simulink library "lib_IronAir"  (R2025b)
settings: Solver=VariableStepAuto  StartTime=0.0  StopTime=10.0  RelTol=1e-3
values from neighbouring files (symbols this model uses):
  IronAir = lib_IronAir_init_params_only()    [generate_mock_cell_curves.m]    (also in lib_IronAir.sldd = 0.01
                        5.0
                    
      ; lib_IronAir_init.m = struct())
undefined symbols (not defined in the file or in its folder): ironair_aggregate_vector, ironair_der_ride_through_vector, ironair_plant_schedule_vector, ironair_sl_cell_dydt, ironair_sl_cell_out, ironair_sl_cell_y0, ironair_sl_electrolyte_dydt, ironair_sl_h2_dydt, ironair_sl_h2_out, ironair_sl_metal_dydt, ironair_sl_metal_out, ironair_sl_oer_out, ironair_sl_orr_dydt, ironair_sl_orr_eta, ironair_sl_thermal_dydt, ironair_standards_assert_vector
settings Model: Creator=admin  LastModifiedBy=admin

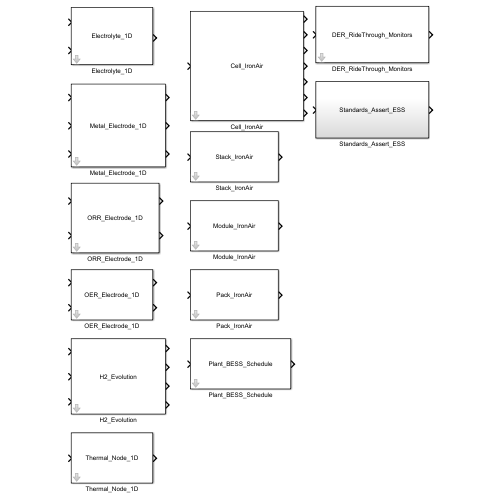
[thumbnail: Simulink's stored preview of the top-level diagram]
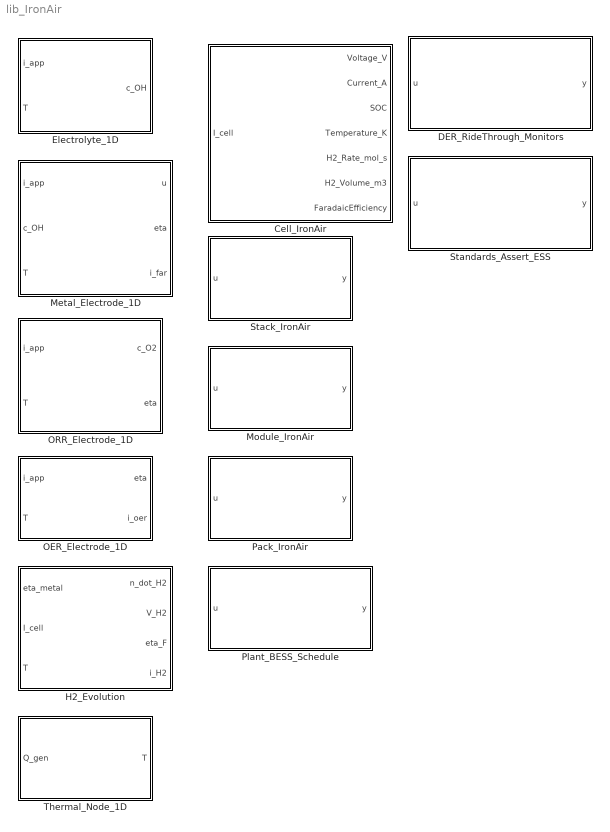
== system lib_IronAir ==
  Cell_IronAir : Subsystem  mask(IronAir){}
      mask help: Iron-Air first-order ODE block Cell_IronAir (Integrator + dy/dt). No S-Functions. Requirements: SSS009 IRS001 SRS017
      mask Help:
      | Continuous first-order ODE realization using Simulink Integrator.
      | Requirements: SSS009 IRS001 SRS017
      mask Display: fprintf('Cell_IronAir')
  DER_RideThrough_Monitors : Subsystem  mask(IronAir){}
      mask help: Iron-Air first-order ODE block DER_RideThrough_Monitors (Integrator + dy/dt). No S-Functions. Requirements: SSS012 SRS011 SRS013
      mask Help:
      | Continuous first-order ODE realization using Simulink Integrator.
      | Requirements: SSS012 SRS011 SRS013
      mask Display: fprintf('DER_RideThrough_Monitors')
  Electrolyte_1D : Subsystem  mask(IronAir){}
      mask help: Iron-Air first-order ODE block Electrolyte_1D (Integrator + dy/dt). No S-Functions. Requirements: SSS003 SRS003 SRS017
      mask Help:
      | Continuous first-order ODE realization using Simulink Integrator.
      | Requirements: SSS003 SRS003 SRS017
      mask Display: fprintf('Electrolyte_1D')
  H2_Evolution : Subsystem  mask(IronAir){}
      mask help: Iron-Air first-order ODE block H2_Evolution (Integrator + dy/dt). No S-Functions. Requirements: SSS007 SRS004 SRS017
      mask Help:
      | Continuous first-order ODE realization using Simulink Integrator.
      | Requirements: SSS007 SRS004 SRS017
      mask Display: fprintf('H2_Evolution')
  Metal_Electrode_1D : Subsystem  mask(IronAir){}
      mask help: Iron-Air first-order ODE block Metal_Electrode_1D (Integrator + dy/dt). No S-Functions. Requirements: SSS004 SRS002 SRS017
      mask Help:
      | Continuous first-order ODE realization using Simulink Integrator.
      | Requirements: SSS004 SRS002 SRS017
      mask Display: fprintf('Metal_Electrode_1D')
  Module_IronAir : Subsystem  mask(IronAir){}
      mask help: Iron-Air first-order ODE block Module_IronAir (Integrator + dy/dt). No S-Functions. Requirements: SSS010
      mask Help:
      | Continuous first-order ODE realization using Simulink Integrator.
      | Requirements: SSS010
      mask Display: fprintf('Module_IronAir')
  OER_Electrode_1D : Subsystem  mask(IronAir){}
      mask help: Iron-Air first-order ODE block OER_Electrode_1D (Integrator + dy/dt). No S-Functions. Requirements: SSS006 SRS002
      mask Help:
      | Continuous first-order ODE realization using Simulink Integrator.
      | Requirements: SSS006 SRS002
      mask Display: fprintf('OER_Electrode_1D')
  ORR_Electrode_1D : Subsystem  mask(IronAir){}
      mask help: Iron-Air first-order ODE block ORR_Electrode_1D (Integrator + dy/dt). No S-Functions. Requirements: SSS005 SRS002 SRS017
      mask Help:
      | Continuous first-order ODE realization using Simulink Integrator.
      | Requirements: SSS005 SRS002 SRS017
      mask Display: fprintf('ORR_Electrode_1D')
  Pack_IronAir : Subsystem  mask(IronAir){}
      mask help: Iron-Air first-order ODE block Pack_IronAir (Integrator + dy/dt). No S-Functions. Requirements: SSS010 IRS002
      mask Help:
      | Continuous first-order ODE realization using Simulink Integrator.
      | Requirements: SSS010 IRS002
      mask Display: fprintf('Pack_IronAir')
  Plant_BESS_Schedule : Subsystem  mask(IronAir){}
      mask help: Iron-Air first-order ODE block Plant_BESS_Schedule (Integrator + dy/dt). No S-Functions. Requirements: SSS011 SRS006
      mask Help:
      | Continuous first-order ODE realization using Simulink Integrator.
      | Requirements: SSS011 SRS006
      mask Display: fprintf('Plant_BESS_Schedule')
  Stack_IronAir : Subsystem  mask(IronAir){}
      mask help: Iron-Air first-order ODE block Stack_IronAir (Integrator + dy/dt). No S-Functions. Requirements: SSS010
      mask Help:
      | Continuous first-order ODE realization using Simulink Integrator.
      | Requirements: SSS010
      mask Display: fprintf('Stack_IronAir')
  Standards_Assert_ESS : Subsystem  mask(IronAir){}
      mask help: Iron-Air first-order ODE block Standards_Assert_ESS (Integrator + dy/dt). No S-Functions. Requirements: SSS013 SRS012 SRS014 SRS015
      mask Help:
      | Continuous first-order ODE realization using Simulink Integrator.
      | Requirements: SSS013 SRS012 SRS014 SRS015
      mask Display: fprintf('Standards_Assert_ESS')
  Thermal_Node_1D : Subsystem  mask(IronAir){}
      mask help: Iron-Air first-order ODE block Thermal_Node_1D (Integrator + dy/dt). No S-Functions. Requirements: SSS008 SRS007 SRS017
      mask Help:
      | Continuous first-order ODE realization using Simulink Integrator.
      | Requirements: SSS008 SRS007 SRS017
      mask Display: fprintf('Thermal_Node_1D')

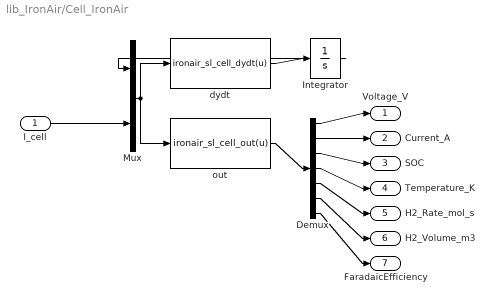
== system lib_IronAir/Cell_IronAir ==
  I_cell : Inport
  Demux : Demux  Outputs=7
  Integrator : Integrator  InitialCondition=ironair_sl_cell_y0()
  Mux : Mux  Inputs=2
  dydt : MATLABFcn  MATLABFcn=ironair_sl_cell_dydt(u)  OutputDimensions=13
  out : MATLABFcn  MATLABFcn=ironair_sl_cell_out(u)  OutputDimensions=7
  Voltage_V : Outport
  Current_A : Outport  Port=2
  SOC : Outport  Port=3
  Temperature_K : Outport  Port=4
  H2_Rate_mol_s : Outport  Port=5
  H2_Volume_m3 : Outport  Port=6
  FaradaicEfficiency : Outport  Port=7
  wires:
  Integrator/1 -> Mux/1
  I_cell/1 -> Mux/2
  Mux/1 -> dydt/1, out/1
  dydt/1 -> Integrator/1
  out/1 -> Demux/1
  Demux/1 -> Voltage_V/1
  Demux/2 -> Current_A/1
  Demux/3 -> SOC/1
  Demux/4 -> Temperature_K/1
  Demux/5 -> H2_Rate_mol_s/1
  Demux/6 -> H2_Volume_m3/1
  Demux/7 -> FaradaicEfficiency/1

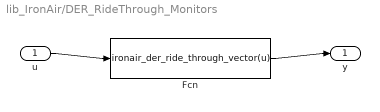
== system lib_IronAir/DER_RideThrough_Monitors ==
  u : Inport
  Fcn : MATLABFcn  MATLABFcn=ironair_der_ride_through_vector(u)  OutputDimensions=3
  y : Outport
  wires:
  u/1 -> Fcn/1
  Fcn/1 -> y/1

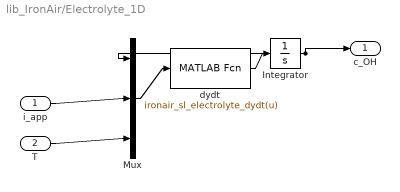
== system lib_IronAir/Electrolyte_1D ==
  i_app : Inport
  T : Inport  Port=2
  Integrator : Integrator  InitialCondition=IronAir.Electrolyte.c_init
  Mux : Mux  Inputs=3
  dydt : MATLABFcn  MATLABFcn=ironair_sl_electrolyte_dydt(u)  OutputDimensions=5
  c_OH : Outport
  wires:
  Integrator/1 -> Mux/1, c_OH/1
  i_app/1 -> Mux/2
  T/1 -> Mux/3
  Mux/1 -> dydt/1
  dydt/1 -> Integrator/1

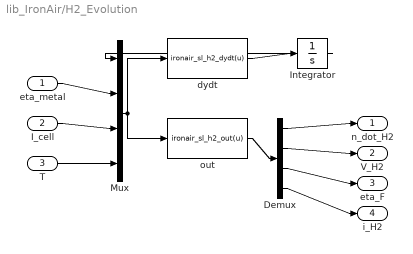
== system lib_IronAir/H2_Evolution ==
  eta_metal : Inport
  I_cell : Inport  Port=2
  T : Inport  Port=3
  Demux : Demux
  Integrator : Integrator
  Mux : Mux
  dydt : MATLABFcn  MATLABFcn=ironair_sl_h2_dydt(u)  OutputDimensions=1
  out : MATLABFcn  MATLABFcn=ironair_sl_h2_out(u)  OutputDimensions=4
  n_dot_H2 : Outport
  V_H2 : Outport  Port=2
  eta_F : Outport  Port=3
  i_H2 : Outport  Port=4
  wires:
  Integrator/1 -> Mux/1
  eta_metal/1 -> Mux/2
  I_cell/1 -> Mux/3
  T/1 -> Mux/4
  Mux/1 -> dydt/1, out/1
  dydt/1 -> Integrator/1
  out/1 -> Demux/1
  Demux/1 -> n_dot_H2/1
  Demux/2 -> V_H2/1
  Demux/3 -> eta_F/1
  Demux/4 -> i_H2/1

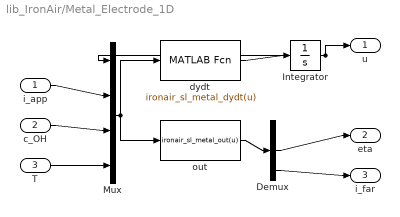
== system lib_IronAir/Metal_Electrode_1D ==
  i_app : Inport
  c_OH : Inport  Port=2
  T : Inport  Port=3
  Demux : Demux  Outputs=3
  Integrator : Integrator  InitialCondition=IronAir.Metal.u_init
  Mux : Mux
  dydt : MATLABFcn  MATLABFcn=ironair_sl_metal_dydt(u)  OutputDimensions=1
  out : MATLABFcn  MATLABFcn=ironair_sl_metal_out(u)  OutputDimensions=3
  u : Outport
  eta : Outport  Port=2
  i_far : Outport  Port=3
  wires:
  Integrator/1 -> Mux/1, u/1
  i_app/1 -> Mux/2
  c_OH/1 -> Mux/3
  T/1 -> Mux/4
  Mux/1 -> dydt/1, out/1
  dydt/1 -> Integrator/1
  out/1 -> Demux/1
  Demux/2 -> eta/1
  Demux/3 -> i_far/1

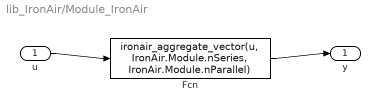
== system lib_IronAir/Module_IronAir ==
  u : Inport
  Fcn : MATLABFcn  MATLABFcn=ironair_aggregate_vector(u, IronAir.Module.nSeries, IronAir.Module.nParallel)  OutputDimensions=8
  y : Outport
  wires:
  u/1 -> Fcn/1
  Fcn/1 -> y/1

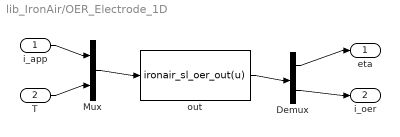
== system lib_IronAir/OER_Electrode_1D ==
  i_app : Inport
  T : Inport  Port=2
  Demux : Demux  Outputs=2
  Mux : Mux  Inputs=2
  out : MATLABFcn  MATLABFcn=ironair_sl_oer_out(u)  OutputDimensions=2
  eta : Outport
  i_oer : Outport  Port=2
  wires:
  i_app/1 -> Mux/1
  T/1 -> Mux/2
  Mux/1 -> out/1
  out/1 -> Demux/1
  Demux/1 -> eta/1
  Demux/2 -> i_oer/1

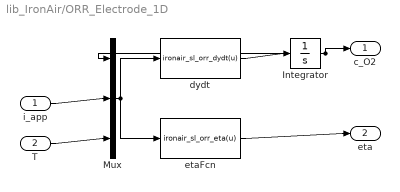
== system lib_IronAir/ORR_Electrode_1D ==
  i_app : Inport
  T : Inport  Port=2
  Integrator : Integrator  InitialCondition=IronAir.ORR.c_init
  Mux : Mux  Inputs=3
  dydt : MATLABFcn  MATLABFcn=ironair_sl_orr_dydt(u)  OutputDimensions=5
  etaFcn : MATLABFcn  MATLABFcn=ironair_sl_orr_eta(u)  OutputDimensions=1
  c_O2 : Outport
  eta : Outport  Port=2
  wires:
  Integrator/1 -> Mux/1, c_O2/1
  i_app/1 -> Mux/2
  T/1 -> Mux/3
  Mux/1 -> dydt/1, etaFcn/1
  dydt/1 -> Integrator/1
  etaFcn/1 -> eta/1

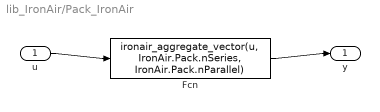
== system lib_IronAir/Pack_IronAir ==
  u : Inport
  Fcn : MATLABFcn  MATLABFcn=ironair_aggregate_vector(u, IronAir.Pack.nSeries, IronAir.Pack.nParallel)  OutputDimensions=8
  y : Outport
  wires:
  u/1 -> Fcn/1
  Fcn/1 -> y/1

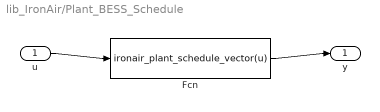
== system lib_IronAir/Plant_BESS_Schedule ==
  u : Inport
  Fcn : MATLABFcn  MATLABFcn=ironair_plant_schedule_vector(u)  OutputDimensions=2
  y : Outport
  wires:
  u/1 -> Fcn/1
  Fcn/1 -> y/1

== system lib_IronAir/Stack_IronAir ==
  u : Inport
  Fcn : MATLABFcn  MATLABFcn=ironair_aggregate_vector(u, IronAir.Stack.nSeries, IronAir.Stack.nParallel)  OutputDimensions=8
  y : Outport
  wires:
  u/1 -> Fcn/1
  Fcn/1 -> y/1

== system lib_IronAir/Standards_Assert_ESS ==
  u : Inport
  Fcn : MATLABFcn  MATLABFcn=ironair_standards_assert_vector(u)  OutputDimensions=4
  y : Outport
  wires:
  u/1 -> Fcn/1
  Fcn/1 -> y/1

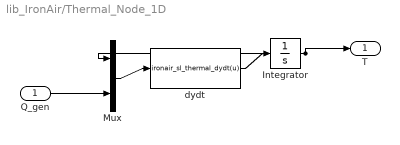
== system lib_IronAir/Thermal_Node_1D ==
  Q_gen : Inport
  Integrator : Integrator  InitialCondition=IronAir.Thermal.T_init
  Mux : Mux  Inputs=2
  dydt : MATLABFcn  MATLABFcn=ironair_sl_thermal_dydt(u)  OutputDimensions=1
  T : Outport
  wires:
  Integrator/1 -> Mux/1, T/1
  Q_gen/1 -> Mux/2
  Mux/1 -> dydt/1
  dydt/1 -> Integrator/1
